simulink model "cllc_plant"  (R2020b)
settings: Solver=FixedStepDiscrete  StartTime=0.0  StopTime=Inf  FixedStep=stepsize  RelTol=1e-3  EnableMultiTasking=on
values from neighbouring files (symbols this model uses):
  Lm1 = Ln*LrP1    (= 0.00016)    [CLLC_Plant_Parameters.m]
  n = 20.0/9.0    (= 2.22222222222)    [CLLC_Plant_Parameters.m]
  stepsize = 2.0E-7    [cllc_data_lib.sldd]
  var_dir_v2g = 0.0    [cllc_data_lib.sldd]
  var_ref_iout = 18.5    [cllc_data_lib.sldd]
  var_ref_vout = 250.0    [cllc_data_lib.sldd]
libraries: fl_lib x219, ee_lib x151, nesl_utility x117, powerlib_meascontrol x15, eeStairGenerator x1
(part 2 of 8)

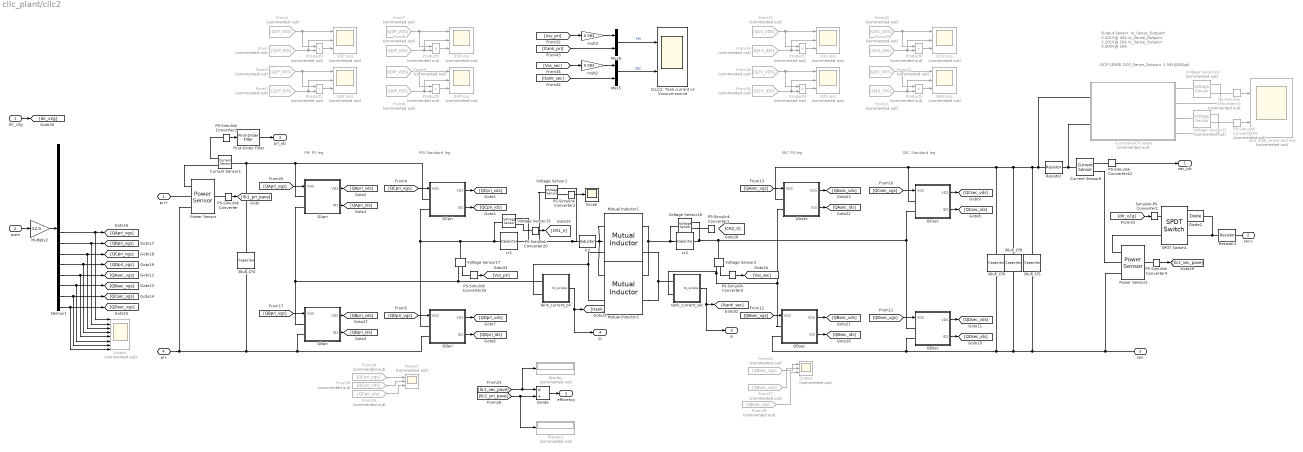
== system cllc_plant/cllc2 ==
  note: OCP SENSE
      |
      | OCP_Sense_Output= 1.59V@50Apk
  note: Output Sensor:
      | Io_Sense_Output= 2.401V@ 40A
      | Io_Sense_Output= 1.201V@ 20A
      | Io_Sense_Output= 0.600V@ 10A
  note: SEC Standard leg
  note: SEC PS leg
  note: PRI PS leg
  note: PRI Standard leg
  dir_v2g : Inport
  pwm : Inport  Port=2
  30uF_Cf1 : fl_lib/Electrical/Electrical Elements/Capacitor  c=18 uF  r=6.5e-3 Ohm  g=0 1/Ohm  i_specify=off  i_priority=None  i=0 A  i_nominal_specify=off  i_nominal_unit=A  i_nominal_value=1  v_specify=off  v_priority=None  v=0.1 V  v_nominal_specify=off  v_nominal_unit=V  v_nominal_value=1  vc_specify=on  vc_priority=High  vc=1 V  vc_nominal_specify=off  vc_nominal_unit=V  vc_nominal_value=1
  30uF_Cf4 : fl_lib/Electrical/Electrical Elements/Capacitor  c=235 nF  r=1.08e-3 Ohm  g=0 1/Ohm  i_specify=off  i_priority=None  i=0 A  i_nominal_specify=off  i_nominal_unit=A  i_nominal_value=1  v_specify=off  v_priority=None  v=0 V  v_nominal_specify=off  v_nominal_unit=V  v_nominal_value=1  vc_specify=off  vc_priority=High  vc=0 V  vc_nominal_specify=off  vc_nominal_unit=V  vc_nominal_value=1
  30uF_Cf6 : fl_lib/Electrical/Electrical Elements/Capacitor  c=250 nF  r=1.08e-3 Ohm  g=0 1/Ohm  i_specify=off  i_priority=None  i=0 A  i_nominal_specify=off  i_nominal_unit=A  i_nominal_value=1  v_specify=off  v_priority=None  v=0.1 V  v_nominal_specify=off  v_nominal_unit=V  v_nominal_value=1  vc_specify=on  vc_priority=High  vc=1 V  vc_nominal_specify=off  vc_nominal_unit=V  vc_nominal_value=1
  30uF_Cf8 : fl_lib/Electrical/Electrical Elements/Capacitor  c=18 uF  r=6.5e-3 Ohm  g=0 1/Ohm  i_specify=off  i_priority=None  i=0 A  i_nominal_specify=off  i_nominal_unit=A  i_nominal_value=1  v_specify=off  v_priority=None  v=0.1 V  v_nominal_specify=off  v_nominal_unit=V  v_nominal_value=1  vc_specify=on  vc_priority=High  vc=1 V  vc_nominal_specify=off  vc_nominal_unit=V  vc_nominal_value=1
  CLLC2: Tank current vs Vsource-source : Scope  NumInputPorts=2
  Current Sensor1 : fl_lib/Electrical/Electrical Sensors/Current Sensor
  Current Sensor8 : fl_lib/Electrical/Electrical Sensors/Current Sensor
  Current+OCP sense : Subsystem  Commented=on
  Demux1 : Demux  Outputs=16
  Diode2 : ee_lib/Semiconductors & Converters/Diode  ModelType=ee.enum.diode.modelType.pwl  IfMat=[.07, .12, .19, 1.75, 4.24, 7.32, 11.2; .16, .3, .72, 2.14, 4.02, 6.35, 9.12] A  TjVec=[25, 125] degC  VfVec=[.5, .7, .9, 1.3, 1.7, 2.1, 2.5] V  Vf=0.6 V  Ron=0.3 Ohm  Goff=1e-8 S  prmExp=ee.enum.diode.expParam.useTwo  I12=[.0137, .545] A  V12=[.6, .7] V  IS=1e-12 A  ec=1  I1=0.0137 A  V1=0.6 V  RS=0 Ohm  Tmeas=25 degC  N_series=1  N_parallel=1  Rz=0.3 Ohm  BV=inf V  C_param=ee.enum.diode.capParam.fixed  CJ=5 pF  CJ0=5 pF  VJ=1 V  Mgrad=0.5  Vvec=[.1, 10, 100] V  Cvec=[3.5, 1, .4] pF  FC=0.5  Q_param=ee.enum.diode.recoveryParam.off  iRM=-7.15 A  iF=4 A  didt=-750 A/us  trr_factor=3  trr=115 ns  Qrr=1500 s*uA  TT=50 ns  tau=100 ns  T_param=ee.enum.diode.temperatureParam.off  IS_T2=1.25e-7 A  I1_T2=0.245 A  V1_T2=0.5 V  Tmeas2=125 degC  EG_param=ee.enum.diode.egapParam.material_si  EG=1.11 eV  XTI_param=ee.enum.diode.xtiParam.pn  XTI=3  dBVdT=0 V/K  Tdevice=25 degC  i_specify=off  i_priority=None  i=0 A  i_nominal_specify=off  i_nominal_unit=A  i_nominal_value=1  v_specify=off  v_priority=None  v=0 V  v_nominal_specify=off  v_nominal_unit=V  v_nominal_value=1  i_capacitor_specify=off  i_capacitor_priority=None  i_capacitor=0 A  i_capacitor_nominal_specify=off  i_capacitor_nominal_unit=A  i_capacitor_nominal_value=1  v_capacitor_specify=off  v_capacitor_priority=None  v_capacitor=0 V  v_capacitor_nominal_specify=off  v_capacitor_nominal_unit=V  v_capacitor_nominal_value=1  power_dissipated_specify=off  power_dissipated_priority=None  power_dissipated=0 W  power_dissipated_nominal_specify=off  power_dissipated_nominal_unit=W  power_dissipated_nominal_value=1  thermal_network_parameterization=ee.enum.thermalNetworkTopology.cauer  Rth=[0, 10] K/W  Rth_Foster=[4, 6] K/W  thermal_mass_parameterization=ee.enum.thermalNetwork.timeconstant  thermal_mass=[0, 1] J/K  thermal_mass_Foster=[1.5, 3] J/K  thermal_time_constant=[0, 10] s  thermal_time_constant_Foster=[6, 18] s  thermal_mass_initial_temperatures=[25, 25] degC
  Display : Display  Commented=on
  Display1 : Display  Commented=on
  Divide : Product  Inputs=*/
  First-Order Filter : powerlib_meascontrol/Filters/First-Order Filter  FilterType=Lowpass  Tc=150e-4  Ts=stepsize  Initialize=off  Vac_Init=[0, 0, 60]  Vdc_Init=0  PlotResponse=off  FreqRange="[0,  200,  1]"
  From : From  Commented=on  GotoTag=Q1P_IDS
  From1 : From  Commented=on  GotoTag=Q1P_VDS
  From14 : From  Commented=on  GotoTag=Q1S_IDS
  From15 : From  Commented=on  GotoTag=Q1S_VDS
  From16 : From  Commented=on  GotoTag=Q2S_IDS
  From18 : From  Commented=on  GotoTag=Q2S_VDS
  From19 : From  Commented=on  GotoTag=Q3S_IDS
  From2 : From  Commented=on  GotoTag=Q2P_IDS
  From20 : From  Commented=on  GotoTag=Q3S_VDS
  From21 : From  Commented=on  GotoTag=Q4S_IDS
  From22 : From  Commented=on  GotoTag=Q4S_VDS
  From24 : From  Commented=on  GotoTag=QBsec_vgs
  From27 : From  Commented=on  GotoTag=QBsec_vds
  From28 : From  Commented=on  GotoTag=QBsec_ids
  From29 : From  Commented=on  GotoTag=QCpri_vgs
  From3 : From  Commented=on  GotoTag=Q2P_VDS
  From30 : From  Commented=on  GotoTag=QCpri_vds
  From31 : From  Commented=on  GotoTag=QCpri_ids
  From6 : From  Commented=on  GotoTag=Q3P_IDS
  From7 : From  Commented=on  GotoTag=Q3P_VDS
  From8 : From  Commented=on  GotoTag=Q4P_IDS
  From9 : From  Commented=on  GotoTag=Q4P_VDS
  Multiply2 : Gain  Gain=12.5  OutDataTypeStr=double
  Mutual Inductor1 : ee_lib/Passive/Transformers/Mutual Inductor  L1=67.5e-6 H  L2=67.5e-6/(0.8*0.8) H  k=0.999  L_tol=5  enable_L1_tol=0  L1_tol_distribution=1  L1_nSigma=4  enable_L2_tol=0  L2_tol_distribution=1  L2_nSigma=4  r=[15.292e-3, 14.309e-3] Ohm  g=[1e-09, 1e-09] 1/Ohm  enable_operating_limits=0  operating_limit_action=2  max_working_current=1 A  power_rating=1 W  enable_faults=0  fault_action=1  fault_winding=1  lambdaPercent=50  turnsShort=0  openCct=0  groundShort=0  groundShortG=0 1/Ohm  tau_fault=1e-3 s  enable_temporal_fault=0  t_fault=1 s  enable_behavioral_fault=0  max_permissible_voltage=100 V  n_fail_on_voltage=1  max_permissible_current=1 A  t_fail_on_current=1 s  iL1_specify=off  iL1_priority=High  iL1=0 A  iL1_nominal_specify=off  iL1_nominal_unit=A  iL1_nominal_value=1  iL2_specify=off  iL2_priority=High  iL2=0 A  iL2_nominal_specify=off  iL2_nominal_unit=A  iL2_nominal_value=1
      settings: SourceProductBaseCode=PS  InternalSimscapePortConfiguration="{\"Bottom\":[],\"Left\":[{\"id\":\"p1\",\"label\":\"1+\",\"type\":\"foundation.electrical.electrical\"},{\"id\":\"n1\",\"label\":\"1-\",\"type\":\"foundation.electrical.electrical\"}],\"Right\":[{\"id\":\"p2\",\"label\":\"2+\",\"type\":\"foundation.electrical.electrical\"},{\"id\":\"n2\",\"label\":\"2-\",\"type\":\"foundation.electrical.electrical\"}],\"Top\":[]}"
  Mutual Inductor2 : ee_lib/Passive/Transformers/Mutual Inductor  L1=67.5e-6 H  L2=67.5e-6/(0.8*0.8) H  k=0.999  L_tol=5  enable_L1_tol=0  L1_tol_distribution=1  L1_nSigma=4  enable_L2_tol=0  L2_tol_distribution=1  L2_nSigma=4  r=[15.292e-3, 14.309e-3] Ohm  g=[1e-09, 1e-09] 1/Ohm  enable_operating_limits=0  operating_limit_action=2  max_working_current=1 A  power_rating=1 W  enable_faults=0  fault_action=1  fault_winding=1  lambdaPercent=50  turnsShort=0  openCct=0  groundShort=0  groundShortG=0 1/Ohm  tau_fault=1e-3 s  enable_temporal_fault=0  t_fault=1 s  enable_behavioral_fault=0  max_permissible_voltage=100 V  n_fail_on_voltage=1  max_permissible_current=1 A  t_fail_on_current=1 s  iL1_specify=off  iL1_priority=High  iL1=0 A  iL1_nominal_specify=off  iL1_nominal_unit=A  iL1_nominal_value=1  iL2_specify=off  iL2_priority=High  iL2=0 A  iL2_nominal_specify=off  iL2_nominal_unit=A  iL2_nominal_value=1
      settings: SourceProductBaseCode=PS  InternalSimscapePortConfiguration="{\"Bottom\":[],\"Left\":[{\"id\":\"p1\",\"label\":\"1+\",\"type\":\"foundation.electrical.electrical\"},{\"id\":\"n1\",\"label\":\"1-\",\"type\":\"foundation.electrical.electrical\"}],\"Right\":[{\"id\":\"p2\",\"label\":\"2+\",\"type\":\"foundation.electrical.electrical\"},{\"id\":\"n2\",\"label\":\"2-\",\"type\":\"foundation.electrical.electrical\"}],\"Top\":[]}"
  Mux5 : Mux  Inputs=2
  Mux6 : Mux  Inputs=2
  PS-Simulink Converter : nesl_utility/PS-Simulink Converter  PhysicalDomain=network_engine_domain  SubClassName=ps_output  LeftPortType=input  RightPortType=output  PseudoPeriodic=off  Frequencies=[]  Unit=inherit  AffineConversion=off
  PS-Simulink Converter{1..3,5,20,25,42} (7 alike) : nesl_utility/PS-Simulink Converter  PhysicalDomain=network_engine_domain  SubClassName=ps_output  LeftPortType=input  RightPortType=output  PseudoPeriodic=off  Frequencies=[]  Unit=1  AffineConversion=off
  PS-Simulink Converter33 : nesl_utility/PS-Simulink Converter  Commented=on  PhysicalDomain=network_engine_domain  SubClassName=ps_output  LeftPortType=input  RightPortType=output  PseudoPeriodic=off  Frequencies=[]  Unit=1  AffineConversion=off
  PS-Simulink Converter34 : nesl_utility/PS-Simulink Converter  Commented=on  PhysicalDomain=network_engine_domain  SubClassName=ps_output  LeftPortType=input  RightPortType=output  PseudoPeriodic=off  Frequencies=[]  Unit=1  AffineConversion=off
  PS-Simulink Converter4 : nesl_utility/PS-Simulink Converter  PhysicalDomain=network_engine_domain  SubClassName=ps_output  LeftPortType=input  RightPortType=output  PseudoPeriodic=off  Frequencies=[]  Unit=inherit  AffineConversion=off
  Power Sensor : ee_lib/Sensors & Transducers/Power Sensor  measurement_type=2  averaging_period=1e-4 s
      settings: SourceProductBaseCode=PS
  Power Sensor1 : ee_lib/Sensors & Transducers/Power Sensor  measurement_type=2  averaging_period=1e-4 s
      settings: SourceProductBaseCode=PS
  Product{1..7,9} (8 alike) : Product  Commented=on
  Q1P loss : Scope  Commented=on  NumInputPorts=3
  Q1S loss : Scope  Commented=on  NumInputPorts=3
  Q2P loss : Scope  Commented=on  NumInputPorts=3
  Q2S loss : Scope  Commented=on  NumInputPorts=3
  Q3P loss : Scope  Commented=on  NumInputPorts=3
  Q3S loss : Scope  Commented=on  NumInputPorts=3
  Q4P loss : Scope  Commented=on  NumInputPorts=3
  Q4S loss : Scope  Commented=on  NumInputPorts=3
  QApri : Subsystem
  QAsec : Subsystem
  QBpri : Subsystem
  QBsec : Subsystem
  QCpri : Subsystem
  QCsec : Subsystem
  QDpri : Subsystem
  QDsec : Subsystem
  Resistor : ee_lib/Passive/Resistor  R=0.001 Ohm  R_tol=5  enable_R_tol=0  tol_distribution=1  nSigma=4  enable_operating_limits=0  operating_limit_action=2  max_working_voltage=100 V  power_rating=1 W  enable_faults=0  fault_action=1  R_faulted=inf Ohm  enable_temporal_fault=0  t_fault=1 s  enable_behavioral_fault=0  max_permissible_current=1 A  t_fail_on_current=1 s  noise_mode=0  sample_time=1e-3 s  repeatability=1  auto_seed=2813624503  user_seed=0  Tdevice=25 degC  alpha=3.93e-3 1/K  Tmeas=25 degC  thermal_mass=100 J/K  power_derating_T1=70 degC  power_derating_T2=155 degC  operating_temperature_range_vec=[-50, 150] degC  temperature_specify=off  temperature_priority=High  temperature=298.15 K  temperature_nominal_specify=off  temperature_nominal_unit=K  temperature_nominal_value=1
  Resistor1 : ee_lib/Passive/Resistor  R=10 Ohm  R_tol=5  enable_R_tol=0  tol_distribution=1  nSigma=4  enable_operating_limits=0  operating_limit_action=2  max_working_voltage=100 V  power_rating=1 W  enable_faults=0  fault_action=1  R_faulted=inf Ohm  enable_temporal_fault=0  t_fault=1 s  enable_behavioral_fault=0  max_permissible_current=1 A  t_fail_on_current=1 s  noise_mode=0  sample_time=1e-3 s  repeatability=1  auto_seed=418932850  user_seed=0  Tdevice=25 degC  alpha=3.93e-3 1/K  Tmeas=25 degC  thermal_mass=100 J/K  power_derating_T1=70 degC  power_derating_T2=155 degC  operating_temperature_range_vec=[-50, 150] degC  temperature_specify=off  temperature_priority=High  temperature=298.15 K  temperature_nominal_specify=off  temperature_nominal_unit=K  temperature_nominal_value=1
  SPDT Switch1 : ee_lib/Switches & Breakers/SPDT Switch  R_closed=1e-3 Ohm  G_open=1e-6 S  Threshold=0.5 V  Width=0 V  model_dynamics=0  t_on=1e-3 s  t_off=1e-3 s  initial_vT=0 V
      settings: SourceProductBaseCode=PS
  Scope : Scope
  Scope1 : Scope  Commented=on  NumInputPorts=8
  Scope2 : Scope  Commented=on  NumInputPorts=3
  Scope3 : Scope  Commented=on  NumInputPorts=3
  Simulink-PS Converter1 : nesl_utility/Simulink-PS Converter  PhysicalDomain=network_engine_domain  SubClassName=ps_input  LeftPortType=input  RightPortType=output  PseudoPeriodic=off  Frequencies=[]  NoiseDistribution=none  NoiseParameters=[]  Unit=1  AffineConversion=off  FilteringAndDerivatives=provide  SimscapeFilterOrder=1  InputFilterTimeConstant=0.001  UdotUserProvided=0
  Voltage Sensor{1..2,15,17..18} (5 alike) : fl_lib/Electrical/Electrical Sensors/Voltage Sensor
  Voltage Sensor24 : fl_lib/Electrical/Electrical Sensors/Voltage Sensor  Commented=on
  Voltage Sensor25 : fl_lib/Electrical/Electrical Sensors/Voltage Sensor  Commented=on
  cr1 : fl_lib/Electrical/Electrical Elements/Capacitor  c=160 nF  r=6e-6 Ohm  g=0 1/Ohm  i_specify=off  i_priority=None  i=0 A  i_nominal_specify=off  i_nominal_unit=A  i_nominal_value=1  v_specify=off  v_priority=None  v=0 V  v_nominal_specify=off  v_nominal_unit=V  v_nominal_value=1  vc_specify=off  vc_priority=High  vc=0 V  vc_nominal_specify=off  vc_nominal_unit=V  vc_nominal_value=1
      settings: LogSimulationData=on
  cr2 : fl_lib/Electrical/Electrical Elements/Capacitor  c=160 nF  r=6e-6 Ohm  g=0 1/Ohm  i_specify=off  i_priority=None  i=0 A  i_nominal_specify=off  i_nominal_unit=A  i_nominal_value=1  v_specify=off  v_priority=None  v=0 V  v_nominal_specify=off  v_nominal_unit=V  v_nominal_value=1  vc_specify=off  vc_priority=High  vc=0 V  vc_nominal_specify=off  vc_nominal_unit=V  vc_nominal_value=1
      settings: LogSimulationData=on
  iout_total_sense and ocp : Scope  Commented=on  NumInputPorts=2
  lr2 : ee_lib/Passive/Inductor  l=16e-6 H  L_tol=0.1  enable_L_tol=0  tol_distribution=1  nSigma=4  r=0.65e-3 Ohm  g=1e-9 1/Ohm  enable_operating_limits=0  operating_limit_action=2  max_working_current=1 A  power_rating=1 W  enable_faults=0  fault_action=1  lambdaPercent=50  k_faulted=0.9999  turnsShort=0  openCct=0  groundShort=0  groundShortG=0 1/Ohm  tau_fault=1e-3 s  enable_temporal_fault=0  t_fault=1 s  enable_behavioral_fault=0  max_permissible_voltage=100 V  n_fail_on_voltage=1  max_permissible_current=1 A  t_fail_on_current=1 s  i_L_specify=off  i_L_priority=High  i_L=0.01 A  i_L_nominal_specify=off  i_L_nominal_unit=A  i_L_nominal_value=1
      settings: LogSimulationData=on
  mult2 : Gain  Gain=0.083
  mult3 : Gain  Gain=0.083
  tank_current_pri : Subsystem  Variant=on
  tank_current_sec : Subsystem  Variant=on
  pri+ : PMIOPort  Side=Left
  sec+ : PMIOPort  Port=2  Side=Right
  sec- : PMIOPort  Port=3  Side=Right
  pri- : PMIOPort  Port=4  Side=Left
  sec_idc : Outport
  pri_idc : Outport  Port=2
  is : Outport  Port=3
  ip : Outport  Port=4
  efficiency : Outport  Port=5
  wires:
  PS-Simulink Converter3/1 -> First-Order Filter/1
  From31/1 -> Scope3/3
  From30/1 -> Scope3/2
  From29/1 -> Scope3/1
  From24/1 -> Scope2/1
  From27/1 -> Scope2/2
  From28/1 -> Scope2/3
  Divide/1 -> efficiency/1
  [llc1_pri_pave] -> Divide/2, Display1/1
  [llc1_sec_pave] -> Divide/1, Display/1
  PS-Simulink Converter4/1 -> [llc1_sec_pave]
  PS-Simulink Converter/1 -> [llc1_pri_pave]
  Multiply2/1 -> Demux1/1
  pwm/1 -> Multiply2/1
  PS-Simulink Converter2/1 -> Scope/1
  tank_current_sec/1(to_scope) -> [Itank_sec], is/1
  tank_current_pri/1(to_scope) -> [Itank_pri], ip/1
  PS-Simulink Converter20/1 -> [CR1_V]
  Product7/1 -> Q1S loss/3
  From14/1 -> Q1S loss/2, Product7/2
  From15/1 -> Product7/1, Q1S loss/1
  From18/1 -> Q2S loss/1, Product4/1
  From16/1 -> Product4/2, Q2S loss/2
  Product4/1 -> Q2S loss/3
  Product5/1 -> Q4S loss/3
  From21/1 -> Q4S loss/2, Product5/2
  From22/1 -> Product5/1, Q4S loss/1
  From20/1 -> Q3S loss/1, Product6/1
  From19/1 -> Product6/2, Q3S loss/2
  Product6/1 -> Q3S loss/3
  [QAsec_vgs] -> QAsec/1(VGS)
  QAsec/2(IDS) -> [QAsec_ids]
  QAsec/1(VDS) -> [QAsec_vds]
  QBsec/1(VDS) -> [QBsec_vds]
  QBsec/2(IDS) -> [QBsec_ids]
  [QBsec_vgs] -> QBsec/1(VGS)
  [QDsec_vgs] -> QDsec/1(VGS)
  QDsec/2(IDS) -> [QDsec_ids]
  QDsec/1(VDS) -> [QDsec_vds]
  QCsec/1(VDS) -> [QCsec_vds]
  QCsec/2(IDS) -> [QCsec_ids]
  [QCsec_vgs] -> QCsec/1(VGS)
  PS-Simulink Converter33/1 -> iout_total_sense and ocp/1
  PS-Simulink Converter34/1 -> iout_total_sense and ocp/2
  Product3/1 -> Q3P loss/3
  From6/1 -> Q3P loss/2, Product3/2
  From7/1 -> Product3/1, Q3P loss/1
  From9/1 -> Q4P loss/1, Product2/1
  From8/1 -> Product2/2, Q4P loss/2
  Product2/1 -> Q4P loss/3
  QDpri/1(VDS) -> [QDpri_vds]
  QDpri/2(IDS) -> [QDpri_ids]
  [QDpri_vgs] -> QDpri/1(VGS)
  [QCpri_vgs] -> QCpri/1(VGS)
  QCpri/2(IDS) -> [QCpri_ids]
  QCpri/1(VDS) -> [QCpri_vds]
  Product1/1 -> Q2P loss/3
  From2/1 -> Q2P loss/2, Product1/2
  From3/1 -> Product1/1, Q2P loss/1
  From1/1 -> Q1P loss/1, Product9/1
  From/1 -> Product9/2, Q1P loss/2
  QBpri/2(IDS) -> [QBpri_ids]
  QApri/1(VDS) -> [QApri_vds]
  QApri/2(IDS) -> [QApri_ids]
  Demux1/15 -> [QCsec_vgs], Scope1/7
  Demux1/14 -> [QBsec_vgs], Scope1/6
  Demux1/13 -> [QAsec_vgs], Scope1/5
  Demux1/16 -> [QDsec_vgs], Scope1/8
  Demux1/12 -> [QDpri_vgs], Scope1/4
  Demux1/11 -> [QCpri_vgs], Scope1/3
  Demux1/10 -> [QBpri_vgs], Scope1/2
  Demux1/9 -> [QApri_vgs], Scope1/1
  [QApri_vgs] -> QApri/1(VGS)
  [QBpri_vgs] -> QBpri/1(VGS)
  PS-Simulink Converter42/1 -> sec_idc/1
  QBpri/1(VDS) -> [QBpri_vds]
  Product9/1 -> Q1P loss/3
  First-Order Filter/1 -> pri_idc/1
  [dir_v2g] -> Simulink-PS Converter1/1
  dir_v2g/1 -> [dir_v2g]
  [Vss_pri] -> mult3/1
  [Itank_sec] -> Mux5/2
  [Itank_pri] -> Mux6/2
  mult2/1 -> Mux5/1
  Mux6/1 -> CLLC2: Tank current vs Vsource-source/1  "PRI"
  [Vss_sec] -> mult2/1
  mult3/1 -> Mux6/1
  Mux5/1 -> CLLC2: Tank current vs Vsource-source/2  "SEC"
  PS-Simulink Converter5/1 -> [Vss_sec]
  PS-Simulink Converter25/1 -> [Vss_pri]
  connections:
  QApri/LConn1 -- 30uF_Cf4/LConn1 -- Current Sensor1/LConn1 -- QCpri/LConn1
  Mutual Inductor1/LConn1 -- Mutual Inductor2/LConn1 -- lr2/RConn1
  lr2/LConn1 -- Voltage Sensor1/LConn1 -- cr1/RConn1 -- Voltage Sensor15/RConn2 -- Voltage Sensor1/RConn2
  Mutual Inductor1/RConn1 -- Voltage Sensor18/LConn1 -- cr2/LConn1 -- Mutual Inductor2/RConn1
  PS-Simulink Converter4/LConn1 -- Power Sensor1/RConn1
  PS-Simulink Converter/LConn1 -- Power Sensor/RConn1
  PS-Simulink Converter3/LConn1 -- Current Sensor1/RConn1
  Power Sensor/LConn2 -- pri+/RConn1
  Voltage Sensor1/RConn1 -- PS-Simulink Converter2/LConn1
  Voltage Sensor18/RConn1 -- PS-Simulink Converter1/LConn1
  Current+OCP sense/RConn3 -- Voltage Sensor25/LConn1
  Current+OCP sense/RConn4 -- Voltage Sensor25/RConn2
  Current+OCP sense/RConn1 -- Voltage Sensor24/LConn1
  PS-Simulink Converter33/LConn1 -- Voltage Sensor24/RConn1
  PS-Simulink Converter34/LConn1 -- Voltage Sensor25/RConn1
  Current+OCP sense/RConn2 -- Voltage Sensor24/RConn2
  QBpri/LConn1 -- tank_current_pri/LConn1 -- Voltage Sensor17/RConn2 -- QApri/LConn2
  Current Sensor8/RConn2 -- Power Sensor1/LConn2
  QAsec/LConn1 -- 30uF_Cf1/LConn1 -- Resistor/LConn1 -- Current+OCP sense/LConn1 -- 30uF_Cf8/LConn1 -- 30uF_Cf6/LConn1 -- QCsec/LConn1
  PS-Simulink Converter42/LConn1 -- Current Sensor8/RConn1
  Resistor/RConn1 -- Current Sensor8/LConn1 -- Current+OCP sense/LConn2
  Mutual Inductor1/LConn2 -- Mutual Inductor2/LConn2 -- tank_current_pri/LConn2
  Power Sensor1/LConn3 -- 30uF_Cf1/RConn1 -- 30uF_Cf8/RConn1 -- 30uF_Cf6/RConn1 -- QDsec/LConn2 -- QBsec/LConn2 -- sec-/RConn1
  QDpri/LConn1 -- Voltage Sensor17/LConn1 -- cr1/LConn1 -- Voltage Sensor15/LConn1 -- QCpri/LConn2
  Mutual Inductor1/RConn2 -- tank_current_sec/LConn1 -- Mutual Inductor2/RConn2
  PS-Simulink Converter20/LConn1 -- Voltage Sensor15/RConn1
  QDpri/LConn2 -- QBpri/LConn2 -- 30uF_Cf4/RConn1 -- Power Sensor/LConn3 -- pri-/RConn1
  SPDT Switch1/LConn1 -- Simulink-PS Converter1/RConn1
  Resistor1/LConn1 -- Diode2/RConn1 -- SPDT Switch1/RConn2
  Current Sensor1/RConn2 -- Power Sensor/LConn1
  Power Sensor1/LConn1 -- SPDT Switch1/LConn2
  SPDT Switch1/RConn1 -- Diode2/LConn1
  Resistor1/RConn1 -- sec+/RConn1
  Voltage Sensor17/RConn1 -- PS-Simulink Converter25/LConn1
  Voltage Sensor2/RConn1 -- PS-Simulink Converter5/LConn1
  Voltage Sensor18/RConn2 -- cr2/RConn1 -- QDsec/LConn1 -- QCsec/LConn2 -- Voltage Sensor2/LConn1
  QBsec/LConn1 -- Voltage Sensor2/RConn2 -- tank_current_sec/LConn2 -- QAsec/LConn2
